simulink model "transferfn_tuning"  (R2019a)
settings: Solver=VariableStepAuto  StartTime=0.0  StopTime=10.0  RelTol=1e-3
settings Model: Creator=jwats  LastModifiedBy=jwats

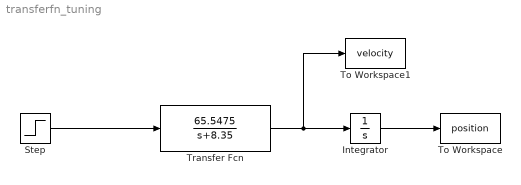
== system transferfn_tuning ==
  Integrator : Integrator
  Step : Step  SampleTime=0
  To Workspace : ToWorkspace  VariableName=position  SaveFormat=Timeseries  SampleTime=-1
  To Workspace1 : ToWorkspace  VariableName=velocity  SaveFormat=Timeseries  SampleTime=-1
  Transfer Fcn : TransferFcn  Numerator=[65.5475]  Denominator=[1 8.35]
  wires:
  Step/1 -> Transfer Fcn/1
  Transfer Fcn/1 -> To Workspace1/1, Integrator/1
  Integrator/1 -> To Workspace/1
